simulink library "HEMERO"  (Simulink 3.00)
values from neighbouring files (symbols this model uses):
  K1 = 0.5    [ejh64.m]    (also in ejh65.m)
  K2 = 0.8    [ejh64.m]    (also in ejh65.m)
  x_camino = 0:0.01:10    [ejh64.m]    (also in ejh65.m)
  y_camino = x_camino.^2    [ejh64.m]    (also in ejh65.m)
undefined symbols (not defined in the file or in its folder): magnitude, nonlinear
libraries: simulink_extras x12, HEMERO x9, simulink3 x6, dspstat x4
(part 7 of 9)

== system HEMERO/Robots móviles/Control de robots móviles/Métodos basados en Teoría de Control/Seguimiento de caminos/Seguimiento de caminos (control no lineal)/Cálculo de parámetros/Cálculo de phi gorro/Subsystem2 ==
  fi_gorro : Inport  Port=1  PortWidth=-1  SampleTime=-1  DataType=auto
      settings: SignalType=auto
  Constant1 : Constant  Value=360
  Constant2 : Constant  Value=360
  Sum1 : Sum  Inputs=-+  SaturateOnIntegerOverflow=on
  Sum2 : Sum  Inputs=++  SaturateOnIntegerOverflow=on
  Switch : Switch  Threshold=180
  Switch1 : Switch  Threshold=0
  Switch2 : Switch  Threshold=-180
  fi_go_mo : Outport  Port=1
  wires:
  Constant2/1 -> Sum2/2
  fi_gorro/1 -> Sum2/1, Switch2/2, Switch2/1, Switch/2, Switch/3, Switch1/2, Sum1/2
  Sum2/1 -> Switch2/3
  Sum1/1 -> Switch/1
  Constant1/1 -> Sum1/1
  Switch2/1 -> Switch1/3
  Switch/1 -> Switch1/1
  Switch1/1 -> fi_go_mo/1

== system HEMERO/Robots móviles/Control de robots móviles/Métodos basados en Teoría de Control/Seguimiento de caminos/Seguimiento de caminos (control no lineal)/Cálculo de parámetros/Subsystem/Parametros de Curvatura ==
  x_1 : Inport  Port=1  PortWidth=-1  SampleTime=-1  DataType=auto
      settings: SignalType=auto
  x_2 : Inport  Port=2  PortWidth=-1  SampleTime=-1  DataType=auto
      settings: SignalType=auto
  x_3 : Inport  Port=3  PortWidth=-1  SampleTime=-1  DataType=auto
      settings: SignalType=auto
  y_1 : Inport  Port=4  PortWidth=-1  SampleTime=-1  DataType=auto
      settings: SignalType=auto
  y_2 : Inport  Port=5  PortWidth=-1  SampleTime=-1  DataType=auto
      settings: SignalType=auto
  y_3 : Inport  Port=6  PortWidth=-1  SampleTime=-1  DataType=auto
      settings: SignalType=auto
  Radio de  Curvatura : Subsystem
  coordenada x c. curvatura : Subsystem
  coordenada y c. curvatura : Subsystem
  x_g : Outport  Port=1  InitialOutput=0
  y_g : Outport  Port=2  InitialOutput=0
  R_c : Outport  Port=3  InitialOutput=0
  wires:
  y_3/1 -> coordenada x c. curvatura/6(y_3), coordenada y c. curvatura/6(y_3)
  y_2/1 -> coordenada y c. curvatura/5(y_2), coordenada x c. curvatura/5(y_2)
  y_1/1 -> Radio de  Curvatura/4(y_1), coordenada x c. curvatura/4(y_1), coordenada y c. curvatura/4(y_1)
  x_3/1 -> coordenada y c. curvatura/3(x_3), coordenada x c. curvatura/3(x_3)
  x_2/1 -> coordenada y c. curvatura/2(x_2), coordenada x c. curvatura/2(x_2)
  x_1/1 -> Radio de  Curvatura/2(x_1), coordenada y c. curvatura/1(x_1), coordenada x c. curvatura/1(x_1)
  coordenada x c. curvatura/1(x_g) -> Radio de  Curvatura/1(x_g), x_g/1
  coordenada y c. curvatura/1(y_g) -> Radio de  Curvatura/3(y_g), y_g/1
  Radio de  Curvatura/1(R_c) -> R_c/1

== system HEMERO/Robots móviles/Control de robots móviles/Métodos basados en Teoría de Control/Seguimiento de caminos/Seguimiento de caminos (control no lineal)/Cálculo de parámetros/Subsystem/Subsystem ==
  x : Inport  Port=1  PortWidth=-1  SampleTime=-1  DataType=auto
      settings: SignalType=auto
  y : Inport  Port=2  PortWidth=-1  SampleTime=-1  DataType=auto
      settings: SignalType=auto
  x_g : Inport  Port=3  PortWidth=-1  SampleTime=-1  DataType=auto
      settings: SignalType=auto
  y_g : Inport  Port=4  PortWidth=-1  SampleTime=-1  DataType=auto
      settings: SignalType=auto
  Math Function2 : Math  Operator=sqrt  OutputSignalType=auto
  Math Function3 : Math  Operator=square  OutputSignalType=auto
  Math Function4 : Math  Operator=square  OutputSignalType=auto
  Sum : Sum  Inputs=+-  SaturateOnIntegerOverflow=on
  Sum1 : Sum  Inputs=+-  SaturateOnIntegerOverflow=on
  Sum2 : Sum  Inputs=++  SaturateOnIntegerOverflow=on
  dist : Outport  Port=1  InitialOutput=0
  wires:
  Sum2/1 -> Math Function2/1
  Math Function4/1 -> Sum2/2
  Sum1/1 -> Math Function4/1
  Math Function3/1 -> Sum2/1
  Sum/1 -> Math Function3/1
  y/1 -> Sum1/1
  x_g/1 -> Sum/2
  x/1 -> Sum/1
  y_g/1 -> Sum1/2
  Math Function2/1 -> dist/1

== system HEMERO/Robots móviles/Control de robots móviles/Métodos basados en Teoría de Control/Seguimiento de caminos/Seguimiento de caminos (control no lineal)/Cálculo de parámetros/Subsystem/distancia mínima1 ==
  x_camino : Inport  Port=1  PortWidth=-1  SampleTime=-1  DataType=auto
      settings: SignalType=auto
  y_camino : Inport  Port=2  PortWidth=-1  SampleTime=-1  DataType=auto
      settings: SignalType=auto
  x_vehiculo : Inport  Port=3  PortWidth=-1  SampleTime=-1  DataType=auto
      settings: SignalType=auto
  y_vehiculo : Inport  Port=4  PortWidth=-1  SampleTime=-1  DataType=auto
      settings: SignalType=auto
  Math Function2 : Math  Operator=sqrt  OutputSignalType=auto
  Math Function3 : Math  Operator=square  OutputSignalType=auto
  Math Function4 : Math  Operator=square  OutputSignalType=auto
  Minimum : dspstat/Minimum
  Sum : Sum  Inputs=+-  SaturateOnIntegerOverflow=on
  Sum1 : Sum  Inputs=+-  SaturateOnIntegerOverflow=on
  Sum2 : Sum  Inputs=++  SaturateOnIntegerOverflow=on
  d_min : Outport  Port=1  InitialOutput=0
  indice : Outport  Port=2  InitialOutput=0
  wires:
  Minimum/2 -> indice/1
  Minimum/1 -> d_min/1
  Math Function2/1 -> Minimum/1
  Sum2/1 -> Math Function2/1
  Math Function4/1 -> Sum2/2
  Sum1/1 -> Math Function4/1
  Math Function3/1 -> Sum2/1
  Sum/1 -> Math Function3/1
  y_vehiculo/1 -> Sum1/2
  y_camino/1 -> Sum1/1
  x_vehiculo/1 -> Sum/2
  x_camino/1 -> Sum/1

== system HEMERO/Robots móviles/Control de robots móviles/Métodos basados en Teoría de Control/Seguimiento de caminos/Seguimiento de caminos (control no lineal)/Cálculo de parámetros/Subsystem/tres_puntos ==
  indice : Inport  Port=1  PortWidth=-1  SampleTime=-1  DataType=auto
      settings: SignalType=auto
  Constant : Constant  Value=1
  Constant1 : Constant  Value=2
  Look-Up Table : Lookup  InputValues=1:length(x_camino)  OutputValues=x_camino(1:length(x_camino))
  Look-Up Table1 : Lookup  InputValues=1:length(y_camino)  OutputValues=y_camino(1:length(y_camino))
  Look-Up Table2 : Lookup  InputValues=1:length(x_camino)  OutputValues=x_camino(1:length(x_camino))
  Look-Up Table3 : Lookup  InputValues=1:length(y_camino)  OutputValues=y_camino(1:length(y_camino))
  Look-Up Table4 : Lookup  InputValues=1:length(x_camino)  OutputValues=x_camino(1:length(x_camino))
  Look-Up Table5 : Lookup  InputValues=1:length(y_camino)  OutputValues=y_camino(1:length(y_camino))
  Sum : Sum  Inputs=++  SaturateOnIntegerOverflow=on
  Sum1 : Sum  Inputs=++  SaturateOnIntegerOverflow=on
  x_1 : Outport  Port=1
  x_2 : Outport  Port=2
  x_3 : Outport  Port=3
  y_1 : Outport  Port=4
  y_2 : Outport  Port=5
  y_3 : Outport  Port=6
  wires:
  Sum1/1 -> Look-Up Table5/1, Look-Up Table4/1
  Look-Up Table4/1 -> x_3/1
  Look-Up Table5/1 -> y_3/1
  Constant1/1 -> Sum1/2
  Look-Up Table1/1 -> y_1/1
  Sum/1 -> Look-Up Table3/1, Look-Up Table2/1
  Look-Up Table3/1 -> y_2/1
  Look-Up Table2/1 -> x_2/1
  Constant/1 -> Sum/2
  indice/1 -> Sum1/1, Sum/1, Look-Up Table1/1, Look-Up Table/1
  Look-Up Table/1 -> x_1/1

== system HEMERO/Robots móviles/Control de robots móviles/Métodos basados en Teoría de Control/Seguimiento de trayectorias/Ejemplos/Ejemplo H.6.6/Seguimiento de trayectorias (Control lineal)/Cambio de variable ==
  x_r : Inport  Port=1  PortWidth=-1  SampleTime=-1  DataType=auto
      settings: SignalType=auto
  x : Inport  Port=2  PortWidth=-1  SampleTime=-1  DataType=auto
      settings: SignalType=auto
  y_r : Inport  Port=3  PortWidth=-1  SampleTime=-1  DataType=auto
      settings: SignalType=auto
  y : Inport  Port=4  PortWidth=-1  SampleTime=-1  DataType=auto
      settings: SignalType=auto
  phi_r : Inport  Port=5  PortWidth=-1  SampleTime=-1  DataType=auto
      settings: SignalType=auto
  phi : Inport  Port=6  PortWidth=-1  SampleTime=-1  DataType=auto
      settings: SignalType=auto
  Cálculo de e1 : Subsystem
  Cálculo de e2 : Subsystem
  Cálculo de e3 : Subsystem
  e1 : Outport  Port=1
  e2 : Outport  Port=2
  e3 : Outport  Port=3
  wires:
  x_r/1 -> Cálculo de e1/1(x_r), Cálculo de e2/1(x_r)
  x/1 -> Cálculo de e1/2(x), Cálculo de e2/2(x)
  y_r/1 -> Cálculo de e1/3(y_r), Cálculo de e2/3(y_r)
  y/1 -> Cálculo de e1/4(y), Cálculo de e2/4(y)
  phi_r/1 -> Cálculo de e3/1(phi_r)
  phi/1 -> Cálculo de e2/5(phi), Cálculo de e3/2(phi), Cálculo de e1/5(phi)
  Cálculo de e1/1(e1) -> e1/1
  Cálculo de e2/1(e2) -> e2/1
  Cálculo de e3/1(e3) -> e3/1

== system HEMERO/Robots móviles/Control de robots móviles/Métodos basados en Teoría de Control/Seguimiento de trayectorias/Ejemplos/Ejemplo H.6.6/Seguimiento de trayectorias (Control lineal)/Configuración síncrona referencia ==
  v_r : Inport  Port=1  PortWidth=-1  SampleTime=-1  DataType=auto
      settings: SignalType=auto
  w_r : Inport  Port=2  PortWidth=-1  SampleTime=-1  DataType=auto
      settings: SignalType=auto
  Gain : Gain  Gain=-1  SaturateOnIntegerOverflow=on
  Integrator : Integrator  ExternalReset=none  InitialConditionSource=internal  InitialCondition=phi_r_inicial  LimitOutput=off  UpperSaturationLimit=inf  LowerSaturationLimit=-inf  ShowSaturationPort=off  ShowStatePort=off  AbsoluteTolerance=auto
  Integrator1 : Integrator  ExternalReset=none  InitialConditionSource=internal  InitialCondition=x_r_inicial  LimitOutput=off  UpperSaturationLimit=inf  LowerSaturationLimit=-inf  ShowSaturationPort=off  ShowStatePort=off  AbsoluteTolerance=auto
  Integrator2 : Integrator  ExternalReset=none  InitialConditionSource=internal  InitialCondition=y_r_inicial  LimitOutput=off  UpperSaturationLimit=inf  LowerSaturationLimit=-inf  ShowSaturationPort=off  ShowStatePort=off  AbsoluteTolerance=auto
  Product : Product  Inputs=2  SaturateOnIntegerOverflow=on
  Product1 : Product  Inputs=2  SaturateOnIntegerOverflow=on
  Trigonometric Function : Trigonometry  Operator=sin  OutputSignalType=auto
  Trigonometric Function1 : Trigonometry  Operator=cos  OutputSignalType=auto
  x_r : Outport  Port=1
  y_r : Outport  Port=2
  phi_r : Outport  Port=3
  wires:
  Product1/1 -> Integrator2/1
  Product/1 -> Integrator1/1
  Trigonometric Function1/1 -> Product1/2
  Integrator/1 -> Trigonometric Function1/1, Trigonometric Function/1, phi_r/1
  Integrator1/1 -> x_r/1
  Integrator2/1 -> y_r/1
  v_r/1 -> Product/1, Product1/1
  w_r/1 -> Integrator/1
  Trigonometric Function/1 -> Gain/1
  Gain/1 -> Product/2

== system HEMERO/Robots móviles/Control de robots móviles/Métodos basados en Teoría de Control/Seguimiento de trayectorias/Ejemplos/Ejemplo H.6.6/Seguimiento de trayectorias (Control lineal)/Configuración síncrona robot real ==
  v : Inport  Port=1  PortWidth=-1  SampleTime=-1  DataType=auto
      settings: SignalType=auto
  w : Inport  Port=2  PortWidth=-1  SampleTime=-1  DataType=auto
      settings: SignalType=auto
  Gain : Gain  Gain=-1  SaturateOnIntegerOverflow=on
  Integrator : Integrator  ExternalReset=none  InitialConditionSource=internal  InitialCondition=phi_inicial  LimitOutput=off  UpperSaturationLimit=inf  LowerSaturationLimit=-inf  ShowSaturationPort=off  ShowStatePort=off  AbsoluteTolerance=auto
  Integrator1 : Integrator  ExternalReset=none  InitialConditionSource=internal  InitialCondition=x_inicial  LimitOutput=off  UpperSaturationLimit=inf  LowerSaturationLimit=-inf  ShowSaturationPort=off  ShowStatePort=off  AbsoluteTolerance=auto
  Integrator2 : Integrator  ExternalReset=none  InitialConditionSource=internal  InitialCondition=y_inicial  LimitOutput=off  UpperSaturationLimit=inf  LowerSaturationLimit=-inf  ShowSaturationPort=off  ShowStatePort=off  AbsoluteTolerance=auto
  Product : Product  Inputs=2  SaturateOnIntegerOverflow=on
  Product1 : Product  Inputs=2  SaturateOnIntegerOverflow=on
  Trigonometric Function : Trigonometry  Operator=sin  OutputSignalType=auto
  Trigonometric Function1 : Trigonometry  Operator=cos  OutputSignalType=auto
  x : Outport  Port=1
  y : Outport  Port=2
  phi : Outport  Port=3
  wires:
  Product1/1 -> Integrator2/1
  Product/1 -> Integrator1/1
  Gain/1 -> Product/2
  Integrator/1 -> Trigonometric Function/1, Trigonometric Function1/1, phi/1
  Integrator1/1 -> x/1
  Integrator2/1 -> y/1
  v/1 -> Product/1, Product1/1
  w/1 -> Integrator/1
  Trigonometric Function/1 -> Gain/1
  Trigonometric Function1/1 -> Product1/2

== system HEMERO/Robots móviles/Control de robots móviles/Métodos basados en Teoría de Control/Seguimiento de trayectorias/Ejemplos/Ejemplo H.6.6/Seguimiento de trayectorias (Control lineal)/Control lineal ==
  e1 : Inport  Port=1  PortWidth=-1  SampleTime=-1  DataType=auto
      settings: SignalType=auto
  e2 : Inport  Port=2  PortWidth=-1  SampleTime=-1  DataType=auto
      settings: SignalType=auto
  e3 : Inport  Port=3  PortWidth=-1  SampleTime=-1  DataType=auto
      settings: SignalType=auto
  v_r : Inport  Port=4  PortWidth=-1  SampleTime=-1  DataType=auto
      settings: SignalType=auto
  Cálculo de u1 : Subsystem
  "Cálculo de u2 " : Subsystem
  u1 : Outport  Port=1
  u2 : Outport  Port=2
  wires:
  e1/1 -> Cálculo de u1/1(e1)
  e2/1 -> "Cálculo de u2 "/1(e2)
  e3/1 -> "Cálculo de u2 "/2(e3)
  Cálculo de u1/1(u1) -> u1/1
  "Cálculo de u2 "/1(u2) -> u2/1
  v_r/1 -> "Cálculo de u2 "/3(v_r)

== system HEMERO/Robots móviles/Control de robots móviles/Métodos basados en Teoría de Control/Seguimiento de trayectorias/Ejemplos/Ejemplo H.6.7/Seguimiento de trayectorias (Control lineal con escalado de velocidad)/Cambio de variable ==
  x_r : Inport  Port=1  PortWidth=-1  SampleTime=-1  DataType=auto
      settings: SignalType=auto
  x : Inport  Port=2  PortWidth=-1  SampleTime=-1  DataType=auto
      settings: SignalType=auto
  y_r : Inport  Port=3  PortWidth=-1  SampleTime=-1  DataType=auto
      settings: SignalType=auto
  y : Inport  Port=4  PortWidth=-1  SampleTime=-1  DataType=auto
      settings: SignalType=auto
  phi_r : Inport  Port=5  PortWidth=-1  SampleTime=-1  DataType=auto
      settings: SignalType=auto
  phi : Inport  Port=6  PortWidth=-1  SampleTime=-1  DataType=auto
      settings: SignalType=auto
  Cálculo de e1 : Subsystem
  Cálculo de e2 : Subsystem
  Cálculo de e3 : Subsystem
  e1 : Outport  Port=1
  e2 : Outport  Port=2
  e3 : Outport  Port=3
  wires:
  x_r/1 -> Cálculo de e1/1(x_r), Cálculo de e2/1(x_r)
  x/1 -> Cálculo de e1/2(x), Cálculo de e2/2(x)
  y_r/1 -> Cálculo de e1/3(y_r), Cálculo de e2/3(y_r)
  y/1 -> Cálculo de e1/4(y), Cálculo de e2/4(y)
  phi_r/1 -> Cálculo de e3/1(phi_r)
  phi/1 -> Cálculo de e2/5(phi), Cálculo de e3/2(phi), Cálculo de e1/5(phi)
  Cálculo de e1/1(e1) -> e1/1
  Cálculo de e2/1(e2) -> e2/1
  Cálculo de e3/1(e3) -> e3/1

== system HEMERO/Robots móviles/Control de robots móviles/Métodos basados en Teoría de Control/Seguimiento de trayectorias/Ejemplos/Ejemplo H.6.7/Seguimiento de trayectorias (Control lineal con escalado de velocidad)/Configuración síncrona referencia ==
  v_r : Inport  Port=1  PortWidth=-1  SampleTime=-1  DataType=auto
      settings: SignalType=auto
  w_r : Inport  Port=2  PortWidth=-1  SampleTime=-1  DataType=auto
      settings: SignalType=auto
  Gain : Gain  Gain=-1  SaturateOnIntegerOverflow=on
  Integrator : Integrator  ExternalReset=none  InitialConditionSource=internal  InitialCondition=phi_r_inicial  LimitOutput=off  UpperSaturationLimit=inf  LowerSaturationLimit=-inf  ShowSaturationPort=off  ShowStatePort=off  AbsoluteTolerance=auto
  Integrator1 : Integrator  ExternalReset=none  InitialConditionSource=internal  InitialCondition=x_r_inicial  LimitOutput=off  UpperSaturationLimit=inf  LowerSaturationLimit=-inf  ShowSaturationPort=off  ShowStatePort=off  AbsoluteTolerance=auto
  Integrator2 : Integrator  ExternalReset=none  InitialConditionSource=internal  InitialCondition=y_r_inicial  LimitOutput=off  UpperSaturationLimit=inf  LowerSaturationLimit=-inf  ShowSaturationPort=off  ShowStatePort=off  AbsoluteTolerance=auto
  Product : Product  Inputs=2  SaturateOnIntegerOverflow=on
  Product1 : Product  Inputs=2  SaturateOnIntegerOverflow=on
  Trigonometric Function : Trigonometry  Operator=sin  OutputSignalType=auto
  Trigonometric Function1 : Trigonometry  Operator=cos  OutputSignalType=auto
  x_r : Outport  Port=1
  y_r : Outport  Port=2
  phi_r : Outport  Port=3
  wires:
  Product1/1 -> Integrator2/1
  Product/1 -> Integrator1/1
  Gain/1 -> Product/2
  Integrator/1 -> Trigonometric Function/1, Trigonometric Function1/1, phi_r/1
  Integrator1/1 -> x_r/1
  Integrator2/1 -> y_r/1
  v_r/1 -> Product/1, Product1/1
  w_r/1 -> Integrator/1
  Trigonometric Function/1 -> Gain/1
  Trigonometric Function1/1 -> Product1/2

== system HEMERO/Robots móviles/Control de robots móviles/Métodos basados en Teoría de Control/Seguimiento de trayectorias/Ejemplos/Ejemplo H.6.7/Seguimiento de trayectorias (Control lineal con escalado de velocidad)/Configuración síncrona robot real ==
  v : Inport  Port=1  PortWidth=-1  SampleTime=-1  DataType=auto
      settings: SignalType=auto
  w : Inport  Port=2  PortWidth=-1  SampleTime=-1  DataType=auto
      settings: SignalType=auto
  Gain : Gain  Gain=-1  SaturateOnIntegerOverflow=on
  Integrator : Integrator  ExternalReset=none  InitialConditionSource=internal  InitialCondition=phi_inicial  LimitOutput=off  UpperSaturationLimit=inf  LowerSaturationLimit=-inf  ShowSaturationPort=off  ShowStatePort=off  AbsoluteTolerance=auto
  Integrator1 : Integrator  ExternalReset=none  InitialConditionSource=internal  InitialCondition=x_inicial  LimitOutput=off  UpperSaturationLimit=inf  LowerSaturationLimit=-inf  ShowSaturationPort=off  ShowStatePort=off  AbsoluteTolerance=auto
  Integrator2 : Integrator  ExternalReset=none  InitialConditionSource=internal  InitialCondition=y_inicial  LimitOutput=off  UpperSaturationLimit=inf  LowerSaturationLimit=-inf  ShowSaturationPort=off  ShowStatePort=off  AbsoluteTolerance=auto
  Product : Product  Inputs=2  SaturateOnIntegerOverflow=on
  Product1 : Product  Inputs=2  SaturateOnIntegerOverflow=on
  Trigonometric Function : Trigonometry  Operator=sin  OutputSignalType=auto
  Trigonometric Function1 : Trigonometry  Operator=cos  OutputSignalType=auto
  x : Outport  Port=1
  y : Outport  Port=2
  phi : Outport  Port=3
  wires:
  Product1/1 -> Integrator2/1
  Product/1 -> Integrator1/1
  Gain/1 -> Product/2
  Integrator/1 -> Trigonometric Function/1, Trigonometric Function1/1, phi/1
  Integrator1/1 -> x/1
  Integrator2/1 -> y/1
  v/1 -> Product/1, Product1/1
  w/1 -> Integrator/1
  Trigonometric Function/1 -> Gain/1
  Trigonometric Function1/1 -> Product1/2

== system HEMERO/Robots móviles/Control de robots móviles/Métodos basados en Teoría de Control/Seguimiento de trayectorias/Ejemplos/Ejemplo H.6.7/Seguimiento de trayectorias (Control lineal con escalado de velocidad)/Control lineal con escalado de velocidad ==
  e1 : Inport  Port=1  PortWidth=-1  SampleTime=-1  DataType=auto
      settings: SignalType=auto
  e2 : Inport  Port=2  PortWidth=-1  SampleTime=-1  DataType=auto
      settings: SignalType=auto
  e3 : Inport  Port=3  PortWidth=-1  SampleTime=-1  DataType=auto
      settings: SignalType=auto
  v_r : Inport  Port=4  PortWidth=-1  SampleTime=-1  DataType=auto
      settings: SignalType=auto
  w_r : Inport  Port=5  PortWidth=-1  SampleTime=-1  DataType=auto
      settings: SignalType=auto
  Cálculo de u1 : Subsystem
  "Cálculo de u2 " : Subsystem
  u1 : Outport  Port=1
  u2 : Outport  Port=2
  wires:
  e1/1 -> Cálculo de u1/1(e1)
  v_r/1 -> Cálculo de u1/2(v_r), "Cálculo de u2 "/3(v_r)
  e2/1 -> "Cálculo de u2 "/1(e2)
  e3/1 -> "Cálculo de u2 "/2(e3)
  Cálculo de u1/1(u1) -> u1/1
  "Cálculo de u2 "/1(u2) -> u2/1
  w_r/1 -> Cálculo de u1/3(w_r)
  Cálculo de u1/2(K1) -> "Cálculo de u2 "/4(K3)

== system HEMERO/Robots móviles/Control de robots móviles/Métodos basados en Teoría de Control/Seguimiento de trayectorias/Ejemplos/Ejemplo H.6.8/Seguimiento de trayectorias (Control no lineal)/Cambio de variable ==
  x_r : Inport  Port=1  PortWidth=-1  SampleTime=-1  DataType=auto
      settings: SignalType=auto
  x : Inport  Port=2  PortWidth=-1  SampleTime=-1  DataType=auto
      settings: SignalType=auto
  y_r : Inport  Port=3  PortWidth=-1  SampleTime=-1  DataType=auto
      settings: SignalType=auto
  y : Inport  Port=4  PortWidth=-1  SampleTime=-1  DataType=auto
      settings: SignalType=auto
  phi_r : Inport  Port=5  PortWidth=-1  SampleTime=-1  DataType=auto
      settings: SignalType=auto
  phi : Inport  Port=6  PortWidth=-1  SampleTime=-1  DataType=auto
      settings: SignalType=auto
  Cálculo de e1 : Subsystem
  Cálculo de e2 : Subsystem
  Cálculo de e3 : Subsystem
  e1 : Outport  Port=1
  e2 : Outport  Port=2
  e3 : Outport  Port=3
  wires:
  x_r/1 -> Cálculo de e1/1(x_r), Cálculo de e2/1(x_r)
  x/1 -> Cálculo de e1/2(x), Cálculo de e2/2(x)
  y_r/1 -> Cálculo de e1/3(y_r), Cálculo de e2/3(y_r)
  y/1 -> Cálculo de e1/4(y), Cálculo de e2/4(y)
  phi_r/1 -> Cálculo de e3/1(phi_r)
  phi/1 -> Cálculo de e2/5(phi), Cálculo de e3/2(phi), Cálculo de e1/5(phi)
  Cálculo de e1/1(e1) -> e1/1
  Cálculo de e2/1(e2) -> e2/1
  Cálculo de e3/1(e3) -> e3/1

== system HEMERO/Robots móviles/Control de robots móviles/Métodos basados en Teoría de Control/Seguimiento de trayectorias/Ejemplos/Ejemplo H.6.8/Seguimiento de trayectorias (Control no lineal)/Configuración síncrona referencia ==
  v_r : Inport  Port=1  PortWidth=-1  SampleTime=-1  DataType=auto
      settings: SignalType=auto
  w_r : Inport  Port=2  PortWidth=-1  SampleTime=-1  DataType=auto
      settings: SignalType=auto
  Gain : Gain  Gain=-1  SaturateOnIntegerOverflow=on
  Integrator : Integrator  ExternalReset=none  InitialConditionSource=internal  InitialCondition=phi_r_inicial  LimitOutput=off  UpperSaturationLimit=inf  LowerSaturationLimit=-inf  ShowSaturationPort=off  ShowStatePort=off  AbsoluteTolerance=auto
  Integrator1 : Integrator  ExternalReset=none  InitialConditionSource=internal  InitialCondition=x_r_inicial  LimitOutput=off  UpperSaturationLimit=inf  LowerSaturationLimit=-inf  ShowSaturationPort=off  ShowStatePort=off  AbsoluteTolerance=auto
  Integrator2 : Integrator  ExternalReset=none  InitialConditionSource=internal  InitialCondition=y_r_inicial  LimitOutput=off  UpperSaturationLimit=inf  LowerSaturationLimit=-inf  ShowSaturationPort=off  ShowStatePort=off  AbsoluteTolerance=auto
  Product : Product  Inputs=2  SaturateOnIntegerOverflow=on
  Product1 : Product  Inputs=2  SaturateOnIntegerOverflow=on
  Trigonometric Function : Trigonometry  Operator=sin  OutputSignalType=auto
  Trigonometric Function1 : Trigonometry  Operator=cos  OutputSignalType=auto
  x_r : Outport  Port=1
  y_r : Outport  Port=2
  phi_r : Outport  Port=3
  wires:
  Product1/1 -> Integrator2/1
  Product/1 -> Integrator1/1
  Integrator/1 -> Trigonometric Function/1, Trigonometric Function1/1, phi_r/1
  Integrator1/1 -> x_r/1
  Integrator2/1 -> y_r/1
  v_r/1 -> Product/1, Product1/1
  w_r/1 -> Integrator/1
  Gain/1 -> Product/2
  Trigonometric Function/1 -> Gain/1
  Trigonometric Function1/1 -> Product1/2

== system HEMERO/Robots móviles/Control de robots móviles/Métodos basados en Teoría de Control/Seguimiento de trayectorias/Ejemplos/Ejemplo H.6.8/Seguimiento de trayectorias (Control no lineal)/Configuración síncrona robot real ==
  v : Inport  Port=1  PortWidth=-1  SampleTime=-1  DataType=auto
      settings: SignalType=auto
  w : Inport  Port=2  PortWidth=-1  SampleTime=-1  DataType=auto
      settings: SignalType=auto
  Gain : Gain  Gain=-1  SaturateOnIntegerOverflow=on
  Integrator : Integrator  ExternalReset=none  InitialConditionSource=internal  InitialCondition=phi_inicial  LimitOutput=off  UpperSaturationLimit=inf  LowerSaturationLimit=-inf  ShowSaturationPort=off  ShowStatePort=off  AbsoluteTolerance=auto
  Integrator1 : Integrator  ExternalReset=none  InitialConditionSource=internal  InitialCondition=x_inicial  LimitOutput=off  UpperSaturationLimit=inf  LowerSaturationLimit=-inf  ShowSaturationPort=off  ShowStatePort=off  AbsoluteTolerance=auto
  Integrator2 : Integrator  ExternalReset=none  InitialConditionSource=internal  InitialCondition=y_inicial  LimitOutput=off  UpperSaturationLimit=inf  LowerSaturationLimit=-inf  ShowSaturationPort=off  ShowStatePort=off  AbsoluteTolerance=auto
  Product : Product  Inputs=2  SaturateOnIntegerOverflow=on
  Product1 : Product  Inputs=2  SaturateOnIntegerOverflow=on
  Trigonometric Function : Trigonometry  Operator=sin  OutputSignalType=auto
  Trigonometric Function1 : Trigonometry  Operator=cos  OutputSignalType=auto
  x : Outport  Port=1
  y : Outport  Port=2
  phi : Outport  Port=3
  wires:
  Product1/1 -> Integrator2/1
  Product/1 -> Integrator1/1
  Gain/1 -> Product/2
  Integrator/1 -> Trigonometric Function/1, Trigonometric Function1/1, phi/1
  Integrator1/1 -> x/1
  Integrator2/1 -> y/1
  v/1 -> Product/1, Product1/1
  w/1 -> Integrator/1
  Trigonometric Function/1 -> Gain/1
  Trigonometric Function1/1 -> Product1/2

== system HEMERO/Robots móviles/Control de robots móviles/Métodos basados en Teoría de Control/Seguimiento de trayectorias/Ejemplos/Ejemplo H.6.8/Seguimiento de trayectorias (Control no lineal)/Control no lineal ==
  e1 : Inport  Port=1  PortWidth=-1  SampleTime=-1  DataType=auto
      settings: SignalType=auto
  e2 : Inport  Port=2  PortWidth=-1  SampleTime=-1  DataType=auto
      settings: SignalType=auto
  e3 : Inport  Port=3  PortWidth=-1  SampleTime=-1  DataType=auto
      settings: SignalType=auto
  v_r : Inport  Port=4  PortWidth=-1  SampleTime=-1  DataType=auto
      settings: SignalType=auto
  K1 : Inport  Port=5  PortWidth=-1  SampleTime=-1  DataType=auto
      settings: SignalType=auto
  K3 : Inport  Port=6  PortWidth=-1  SampleTime=-1  DataType=auto
      settings: SignalType=auto
  Cálculo de u1 : Subsystem
  "Cálculo de u2 " : Subsystem
  u1 : Outport  Port=1
  u2 : Outport  Port=2
  wires:
  e1/1 -> Cálculo de u1/1(e1)
  e2/1 -> "Cálculo de u2 "/1(e2)
  e3/1 -> "Cálculo de u2 "/2(e3)
  Cálculo de u1/1(u1) -> u1/1
  "Cálculo de u2 "/1(u2) -> u2/1
  v_r/1 -> "Cálculo de u2 "/3(v_r)
  K1/1 -> Cálculo de u1/2(K1)
  K3/1 -> "Cálculo de u2 "/4(K3)

== system HEMERO/Robots móviles/Control de robots móviles/Métodos basados en Teoría de Control/Seguimiento de trayectorias/Ejemplos/Ejemplo H.6.8/Seguimiento de trayectorias (Control no lineal)/Cálculo de K1 y K3 ==
  w_r : Inport  Port=1  PortWidth=-1  SampleTime=-1  DataType=auto
      settings: SignalType=auto
  v_r : Inport  Port=2  PortWidth=-1  SampleTime=-1  DataType=auto
      settings: SignalType=auto
  Constant : Constant  Value=b
  Fcn : Fcn  Expr=u^2
  Fcn1 : Fcn  Expr=u^2
  Fcn2 : Fcn  Expr=sqrt(u)
  Gain1 : Gain  Gain=2*d  SaturateOnIntegerOverflow=on
  Product : Product  Inputs=2  SaturateOnIntegerOverflow=on
  Sum : Sum  Inputs=++  SaturateOnIntegerOverflow=on
  K1 : Outport  Port=1
  wires:
  w_r/1 -> Fcn/1
  v_r/1 -> Fcn1/1
  Fcn1/1 -> Product/1
  Constant/1 -> Product/2
  Product/1 -> Sum/1
  Fcn/1 -> Sum/2
  Sum/1 -> Fcn2/1
  Fcn2/1 -> Gain1/1
  Gain1/1 -> K1/1

== system HEMERO/Robots móviles/Control de robots móviles/Métodos basados en Teoría de Control/Seguimiento de trayectorias/Seguimiento de trayectorias (Control lineal con escalado de velocidad)/Cambio de variable/Cálculo de e3/Subsystem2 ==
  phi_gorro : Inport  Port=1  PortWidth=-1  SampleTime=-1  DataType=auto
      settings: SignalType=auto
  Constant1 : Constant  Value=360
  Constant2 : Constant  Value=360
  Sum1 : Sum  Inputs=-+  SaturateOnIntegerOverflow=on
  Sum2 : Sum  Inputs=++  SaturateOnIntegerOverflow=on
  Switch : Switch  Threshold=180
  Switch1 : Switch  Threshold=0
  Switch2 : Switch  Threshold=-180
  phi_go_mod : Outport  Port=1
  wires:
  Constant2/1 -> Sum2/2
  phi_gorro/1 -> Sum2/1, Switch2/2, Switch2/1, Switch/2, Switch/3, Switch1/2, Sum1/2
  Sum2/1 -> Switch2/3
  Sum1/1 -> Switch/1
  Constant1/1 -> Sum1/1
  Switch2/1 -> Switch1/3
  Switch/1 -> Switch1/1
  Switch1/1 -> phi_go_mod/1

== system HEMERO/Robots móviles/Control de robots móviles/Métodos basados en Teoría de Control/Seguimiento de trayectorias/Seguimiento de trayectorias (Control lineal)/Cambio de variable/Cálculo de e3/Subsystem2 ==
  phi_gorro : Inport  Port=1  PortWidth=-1  SampleTime=-1  DataType=auto
      settings: SignalType=auto
  Constant1 : Constant  Value=360
  Constant2 : Constant  Value=360
  Sum1 : Sum  Inputs=-+  SaturateOnIntegerOverflow=on
  Sum2 : Sum  Inputs=++  SaturateOnIntegerOverflow=on
  Switch : Switch  Threshold=180
  Switch1 : Switch  Threshold=0
  Switch2 : Switch  Threshold=-180
  phi_go_mod : Outport  Port=1
  wires:
  Constant2/1 -> Sum2/2
  phi_gorro/1 -> Sum2/1, Switch2/2, Switch2/1, Switch/2, Switch/3, Switch1/2, Sum1/2
  Sum2/1 -> Switch2/3
  Sum1/1 -> Switch/1
  Constant1/1 -> Sum1/1
  Switch2/1 -> Switch1/3
  Switch/1 -> Switch1/1
  Switch1/1 -> phi_go_mod/1

== system HEMERO/Robots móviles/Control de robots móviles/Métodos basados en Teoría de Control/Seguimiento de trayectorias/Seguimiento de trayectorias (Control no lineal)/Cambio de variable/Cálculo de e3/Subsystem2 ==
  phi_gorro : Inport  Port=1  PortWidth=-1  SampleTime=-1  DataType=auto
      settings: SignalType=auto
  Constant1 : Constant  Value=360
  Constant2 : Constant  Value=360
  Sum1 : Sum  Inputs=-+  SaturateOnIntegerOverflow=on
  Sum2 : Sum  Inputs=++  SaturateOnIntegerOverflow=on
  Switch : Switch  Threshold=180
  Switch1 : Switch  Threshold=0
  Switch2 : Switch  Threshold=-180
  phi_go_mod : Outport  Port=1
  wires:
  Constant2/1 -> Sum2/2
  phi_gorro/1 -> Sum2/1, Switch2/2, Switch2/1, Switch/2, Switch/3, Switch1/2, Sum1/2
  Sum2/1 -> Switch2/3
  Sum1/1 -> Switch/1
  Constant1/1 -> Sum1/1
  Switch2/1 -> Switch1/3
  Switch/1 -> Switch1/1
  Switch1/1 -> phi_go_mod/1

== system HEMERO/Robots móviles/Control de robots móviles/Métodos basados en Teoría de Control/Seguimiento de caminos/Ejemplos/Ejemplo H.6.4/Seguimiento de caminos (control lineal)/Cálculo de parámetros/Cálculo de phi gorro ==
  fi_vehiculo : Inport  Port=1  PortWidth=-1  SampleTime=-1  DataType=auto
      settings: SignalType=auto
  indice : Inport  Port=2  PortWidth=-1  SampleTime=-1  DataType=auto
      settings: SignalType=auto
  Subsystem : Subsystem
      mask Type: Pasa phi a un ángulo entre -180 y 180
      mask Description: Pasa phi a un ángulo entre -180 y 180
      mask Help: Pasa phi a un ángulo entre -180 y 180
  Subsystem1 : Subsystem
  Subsystem2 : Subsystem
      mask Description: Pasa phi gorro al intervalo -180,180
  suma : Sum  Inputs=+-  SaturateOnIntegerOverflow=on
  fi_go_mo : Outport  Port=1
  wires:
  Subsystem2/1(fi_go_mo) -> fi_go_mo/1
  suma/1 -> Subsystem2/1(fi_gorro)
  Subsystem/1(fi_veh_mod) -> suma/1
  indice/1 -> Subsystem1/1(indice)
  fi_vehiculo/1 -> Subsystem/1(fi_vehiculo)
  Subsystem1/1(fi_camino) -> suma/2

== system HEMERO/Robots móviles/Control de robots móviles/Métodos basados en Teoría de Control/Seguimiento de caminos/Ejemplos/Ejemplo H.6.4/Seguimiento de caminos (control lineal)/Cálculo de parámetros/Subsystem ==
  x_camino : Inport  Port=1  PortWidth=-1  SampleTime=-1  DataType=auto
      settings: SignalType=auto
  y_camino : Inport  Port=2  PortWidth=-1  SampleTime=-1  DataType=auto
      settings: SignalType=auto
  x_vehiculo : Inport  Port=3  PortWidth=-1  SampleTime=-1  DataType=auto
      settings: SignalType=auto
  y_vehiculo : Inport  Port=4  PortWidth=-1  SampleTime=-1  DataType=auto
      settings: SignalType=auto
  Parametros de Curvatura : Subsystem
  Product : Product  Inputs=2  SaturateOnIntegerOverflow=on
  Rc - dist : Sum  Inputs=-+  SaturateOnIntegerOverflow=on
  Sign : Signum
  Subsystem : Subsystem
  distancia mínima1 : Subsystem
  tres_puntos : Subsystem
  distancia : Outport  Port=1
  indice : Outport  Port=2
  R_c : Outport  Port=3
  wires:
  distancia mínima1/2(indice) -> tres_puntos/1(indice), indice/1
  Parametros de Curvatura/3(R_c) -> R_c/1, Rc - dist/2
  y_vehiculo/1 -> Subsystem/2(y), distancia mínima1/4(y_vehiculo)
  x_vehiculo/1 -> Subsystem/1(x), distancia mínima1/3(x_vehiculo)
  tres_puntos/4(y_1) -> Parametros de Curvatura/4(y_1)
  tres_puntos/1(x_1) -> Parametros de Curvatura/1(x_1)
  Product/1 -> distancia/1
  y_camino/1 -> distancia mínima1/2(y_camino)
  x_camino/1 -> distancia mínima1/1(x_camino)
  tres_puntos/6(y_3) -> Parametros de Curvatura/6(y_3)
  tres_puntos/5(y_2) -> Parametros de Curvatura/5(y_2)
  tres_puntos/3(x_3) -> Parametros de Curvatura/3(x_3)
  tres_puntos/2(x_2) -> Parametros de Curvatura/2(x_2)
  distancia mínima1/1(d_min) -> Product/2
  Sign/1 -> Product/1
  Parametros de Curvatura/1(x_g) -> Subsystem/3(x_g)
  Parametros de Curvatura/2(y_g) -> Subsystem/4(y_g)
  Subsystem/1(dist) -> Rc - dist/1
  Rc - dist/1 -> Sign/1

== system HEMERO/Robots móviles/Control de robots móviles/Métodos basados en Teoría de Control/Seguimiento de caminos/Ejemplos/Ejemplo H.6.5/Seguimiento de caminos (control no lineal)/Cálculo de parámetros/Cálculo de phi gorro ==
  fi_vehiculo : Inport  Port=1  PortWidth=-1  SampleTime=-1  DataType=auto
      settings: SignalType=auto
  indice : Inport  Port=2  PortWidth=-1  SampleTime=-1  DataType=auto
      settings: SignalType=auto
  Subsystem : Subsystem
      mask Type: Pasa phi a un ángulo entre -180 y 180
      mask Description: Pasa phi a un ángulo entre -180 y 180
      mask Help: Pasa phi a un ángulo entre -180 y 180
  Subsystem1 : Subsystem
  Subsystem2 : Subsystem
      mask Description: Pasa phi gorro al intervalo -180,180
  suma : Sum  Inputs=+-  SaturateOnIntegerOverflow=on
  fi_go_mo : Outport  Port=1
  wires:
  Subsystem2/1(fi_go_mo) -> fi_go_mo/1
  suma/1 -> Subsystem2/1(fi_gorro)
  Subsystem/1(fi_veh_mod) -> suma/1
  indice/1 -> Subsystem1/1(indice)
  fi_vehiculo/1 -> Subsystem/1(fi_vehiculo)
  Subsystem1/1(fi_camino) -> suma/2

== system HEMERO/Robots móviles/Control de robots móviles/Métodos basados en Teoría de Control/Seguimiento de caminos/Ejemplos/Ejemplo H.6.5/Seguimiento de caminos (control no lineal)/Cálculo de parámetros/Subsystem ==
  x_camino : Inport  Port=1  PortWidth=-1  SampleTime=-1  DataType=auto
      settings: SignalType=auto
  y_camino : Inport  Port=2  PortWidth=-1  SampleTime=-1  DataType=auto
      settings: SignalType=auto
  x_vehiculo : Inport  Port=3  PortWidth=-1  SampleTime=-1  DataType=auto
      settings: SignalType=auto
  y_vehiculo : Inport  Port=4  PortWidth=-1  SampleTime=-1  DataType=auto
      settings: SignalType=auto
  Parametros de Curvatura : Subsystem
  Product : Product  Inputs=2  SaturateOnIntegerOverflow=on
  Rc - dist : Sum  Inputs=-+  SaturateOnIntegerOverflow=on
  Sign : Signum
  Subsystem : Subsystem
  distancia mínima1 : Subsystem
  tres_puntos : Subsystem
  distancia : Outport  Port=1
  indice : Outport  Port=2
  R_c : Outport  Port=3
  wires:
  distancia mínima1/2(indice) -> tres_puntos/1(indice), indice/1
  Parametros de Curvatura/3(R_c) -> R_c/1, Rc - dist/2
  y_vehiculo/1 -> Subsystem/2(y), distancia mínima1/4(y_vehiculo)
  x_vehiculo/1 -> Subsystem/1(x), distancia mínima1/3(x_vehiculo)
  tres_puntos/4(y_1) -> Parametros de Curvatura/4(y_1)
  tres_puntos/1(x_1) -> Parametros de Curvatura/1(x_1)
  Product/1 -> distancia/1
  y_camino/1 -> distancia mínima1/2(y_camino)
  x_camino/1 -> distancia mínima1/1(x_camino)
  tres_puntos/6(y_3) -> Parametros de Curvatura/6(y_3)
  tres_puntos/5(y_2) -> Parametros de Curvatura/5(y_2)
  tres_puntos/3(x_3) -> Parametros de Curvatura/3(x_3)
  tres_puntos/2(x_2) -> Parametros de Curvatura/2(x_2)
  distancia mínima1/1(d_min) -> Product/2
  Sign/1 -> Product/1
  Parametros de Curvatura/1(x_g) -> Subsystem/3(x_g)
  Parametros de Curvatura/2(y_g) -> Subsystem/4(y_g)
  Subsystem/1(dist) -> Rc - dist/1
  Rc - dist/1 -> Sign/1

== system HEMERO/Robots móviles/Control de robots móviles/Métodos basados en Teoría de Control/Seguimiento de caminos/Seguimiento de caminos (control lineal)/Cálculo de parámetros/Subsystem/Parametros de Curvatura/Radio de  Curvatura ==
  x_g : Inport  Port=1  PortWidth=-1  SampleTime=-1  DataType=auto
      settings: SignalType=auto
  x_1 : Inport  Port=2  PortWidth=-1  SampleTime=-1  DataType=auto
      settings: SignalType=auto
  y_g : Inport  Port=3  PortWidth=-1  SampleTime=-1  DataType=auto
      settings: SignalType=auto
  y_1 : Inport  Port=4  PortWidth=-1  SampleTime=-1  DataType=auto
      settings: SignalType=auto
  Math Function : Math  Operator=square  OutputSignalType=auto
  Math Function1 : Math  Operator=sqrt  OutputSignalType=auto
  Math Function2 : Math  Operator=square  OutputSignalType=auto
  Sum : Sum  Inputs=+-  SaturateOnIntegerOverflow=on
  Sum1 : Sum  Inputs=+-  SaturateOnIntegerOverflow=on
  Sum2 : Sum  Inputs=++  SaturateOnIntegerOverflow=on
  R_c : Outport  Port=1  InitialOutput=0
  wires:
  x_g/1 -> Sum/2
  x_1/1 -> Sum/1
  y_1/1 -> Sum1/1
  y_g/1 -> Sum1/2
  Sum/1 -> Math Function/1
  Sum1/1 -> Math Function2/1
  Math Function/1 -> Sum2/1
  Math Function2/1 -> Sum2/2
  Sum2/1 -> Math Function1/1
  Math Function1/1 -> R_c/1

== system HEMERO/Robots móviles/Control de robots móviles/Métodos basados en Teoría de Control/Seguimiento de caminos/Seguimiento de caminos (control lineal)/Cálculo de parámetros/Subsystem/Parametros de Curvatura/coordenada x c. curvatura ==
  x_1 : Inport  Port=1  PortWidth=-1  SampleTime=-1  DataType=auto
      settings: SignalType=auto
  x_2 : Inport  Port=2  PortWidth=-1  SampleTime=-1  DataType=auto
      settings: SignalType=auto
  x_3 : Inport  Port=3  PortWidth=-1  SampleTime=-1  DataType=auto
      settings: SignalType=auto
  y_1 : Inport  Port=4  PortWidth=-1  SampleTime=-1  DataType=auto
      settings: SignalType=auto
  y_2 : Inport  Port=5  PortWidth=-1  SampleTime=-1  DataType=auto
      settings: SignalType=auto
  y_3 : Inport  Port=6  PortWidth=-1  SampleTime=-1  DataType=auto
      settings: SignalType=auto
  Constant : Constant  Value=0.00000001
  Math Function : Math  Operator=reciprocal  OutputSignalType=auto
  Product{,1..4} (5 alike) : Product  Inputs=2  SaturateOnIntegerOverflow=on
  Sum : Sum  Inputs=+-  SaturateOnIntegerOverflow=on
  Sum1 : Sum  Inputs=+-  SaturateOnIntegerOverflow=on
  Switch : Switch  Threshold=0.00000001
  bloque_1 : Subsystem
  bloque_2 : Subsystem
  x_g : Outport  Port=1  InitialOutput=0
  wires:
  Sum/1 -> Product4/1
  y_3/1 -> bloque_2/4(y3)
  y_2/1 -> bloque_1/4(y2), bloque_2/3(y2)
  x_3/1 -> bloque_2/2(x3)
  y_1/1 -> bloque_1/3(y1)
  x_2/1 -> bloque_2/1(x2), bloque_1/2(x2)
  x_1/1 -> bloque_1/1(x1)
  bloque_2/1(alfa_2) -> Product3/2
  bloque_1/2(beta_1) -> Product3/1, Product1/1
  bloque_1/1(alfa_1) -> Product2/1
  bloque_2/2(beta_2) -> Product2/2, Product/1
  bloque_2/3(c_2) -> Product1/2
  bloque_1/3(c_1) -> Product/2
  Math Function/1 -> Product4/2
  Product3/1 -> Sum1/2
  Product2/1 -> Sum1/1
  Product1/1 -> Sum/2
  Product/1 -> Sum/1
  Product4/1 -> x_g/1
  Sum1/1 -> Switch/2, Switch/1
  Constant/1 -> Switch/3
  Switch/1 -> Math Function/1

== system HEMERO/Robots móviles/Control de robots móviles/Métodos basados en Teoría de Control/Seguimiento de caminos/Seguimiento de caminos (control lineal)/Cálculo de parámetros/Subsystem/Parametros de Curvatura/coordenada y c. curvatura ==
  x_1 : Inport  Port=1  PortWidth=-1  SampleTime=-1  DataType=auto
      settings: SignalType=auto
  x_2 : Inport  Port=2  PortWidth=-1  SampleTime=-1  DataType=auto
      settings: SignalType=auto
  x_3 : Inport  Port=3  PortWidth=-1  SampleTime=-1  DataType=auto
      settings: SignalType=auto
  y_1 : Inport  Port=4  PortWidth=-1  SampleTime=-1  DataType=auto
      settings: SignalType=auto
  y_2 : Inport  Port=5  PortWidth=-1  SampleTime=-1  DataType=auto
      settings: SignalType=auto
  y_3 : Inport  Port=6  PortWidth=-1  SampleTime=-1  DataType=auto
      settings: SignalType=auto
  Constant : Constant  Value=0.00000001
  Math Function : Math  Operator=reciprocal  OutputSignalType=auto
  Product{,1..4} (5 alike) : Product  Inputs=2  SaturateOnIntegerOverflow=on
  Sum : Sum  Inputs=+-  SaturateOnIntegerOverflow=on
  Sum1 : Sum  Inputs=+-  SaturateOnIntegerOverflow=on
  Switch : Switch  Threshold=0.00000001
  bloque_1 : Subsystem
  bloque_2 : Subsystem
  y_g : Outport  Port=1  InitialOutput=0
  wires:
  Sum/1 -> Product4/1
  y_3/1 -> bloque_2/4(y3)
  y_2/1 -> bloque_1/4(y2), bloque_2/3(y2)
  x_3/1 -> bloque_2/2(x3)
  y_1/1 -> bloque_1/3(y1)
  x_2/1 -> bloque_2/1(x2), bloque_1/2(x2)
  x_1/1 -> bloque_1/1(x1)
  Product3/1 -> Sum1/2
  Product2/1 -> Sum1/1
  Product1/1 -> Sum/2
  Product/1 -> Sum/1
  bloque_2/1(alfa_2) -> Product3/1, Product1/2
  bloque_1/2(beta_1) -> Product3/2
  bloque_2/2(beta_2) -> Product2/2
  bloque_1/1(alfa_1) -> Product2/1, Product/1
  bloque_1/3(c_1) -> Product1/1
  bloque_2/3(c_2) -> Product/2
  Product4/1 -> y_g/1
  Math Function/1 -> Product4/2
  Switch/1 -> Math Function/1
  Sum1/1 -> Switch/2, Switch/1
  Constant/1 -> Switch/3

== system HEMERO/Robots móviles/Control de robots móviles/Métodos basados en Teoría de Control/Seguimiento de caminos/Seguimiento de caminos (control no lineal)/Cálculo de parámetros/Subsystem/Parametros de Curvatura/Radio de  Curvatura ==
  x_g : Inport  Port=1  PortWidth=-1  SampleTime=-1  DataType=auto
      settings: SignalType=auto
  x_1 : Inport  Port=2  PortWidth=-1  SampleTime=-1  DataType=auto
      settings: SignalType=auto
  y_g : Inport  Port=3  PortWidth=-1  SampleTime=-1  DataType=auto
      settings: SignalType=auto
  y_1 : Inport  Port=4  PortWidth=-1  SampleTime=-1  DataType=auto
      settings: SignalType=auto
  Math Function : Math  Operator=square  OutputSignalType=auto
  Math Function1 : Math  Operator=sqrt  OutputSignalType=auto
  Math Function2 : Math  Operator=square  OutputSignalType=auto
  Sum : Sum  Inputs=+-  SaturateOnIntegerOverflow=on
  Sum1 : Sum  Inputs=+-  SaturateOnIntegerOverflow=on
  Sum2 : Sum  Inputs=++  SaturateOnIntegerOverflow=on
  R_c : Outport  Port=1  InitialOutput=0
  wires:
  Math Function1/1 -> R_c/1
  Sum2/1 -> Math Function1/1
  Math Function2/1 -> Sum2/2
  Math Function/1 -> Sum2/1
  Sum1/1 -> Math Function2/1
  Sum/1 -> Math Function/1
  y_g/1 -> Sum1/2
  y_1/1 -> Sum1/1
  x_1/1 -> Sum/1
  x_g/1 -> Sum/2

== system HEMERO/Robots móviles/Control de robots móviles/Métodos basados en Teoría de Control/Seguimiento de caminos/Seguimiento de caminos (control no lineal)/Cálculo de parámetros/Subsystem/Parametros de Curvatura/coordenada x c. curvatura ==
  x_1 : Inport  Port=1  PortWidth=-1  SampleTime=-1  DataType=auto
      settings: SignalType=auto
  x_2 : Inport  Port=2  PortWidth=-1  SampleTime=-1  DataType=auto
      settings: SignalType=auto
  x_3 : Inport  Port=3  PortWidth=-1  SampleTime=-1  DataType=auto
      settings: SignalType=auto
  y_1 : Inport  Port=4  PortWidth=-1  SampleTime=-1  DataType=auto
      settings: SignalType=auto
  y_2 : Inport  Port=5  PortWidth=-1  SampleTime=-1  DataType=auto
      settings: SignalType=auto
  y_3 : Inport  Port=6  PortWidth=-1  SampleTime=-1  DataType=auto
      settings: SignalType=auto
  Constant : Constant  Value=0.00000001
  Math Function : Math  Operator=reciprocal  OutputSignalType=auto
  Product{,1..4} (5 alike) : Product  Inputs=2  SaturateOnIntegerOverflow=on
  Sum : Sum  Inputs=+-  SaturateOnIntegerOverflow=on
  Sum1 : Sum  Inputs=+-  SaturateOnIntegerOverflow=on
  Switch : Switch  Threshold=0.00000001
  bloque_1 : Subsystem
  bloque_2 : Subsystem
  x_g : Outport  Port=1  InitialOutput=0
  wires:
  Switch/1 -> Math Function/1
  Constant/1 -> Switch/3
  Sum1/1 -> Switch/1, Switch/2
  Product4/1 -> x_g/1
  Product/1 -> Sum/1
  Product1/1 -> Sum/2
  Product2/1 -> Sum1/1
  Product3/1 -> Sum1/2
  Math Function/1 -> Product4/2
  bloque_1/3(c_1) -> Product/2
  bloque_2/3(c_2) -> Product1/2
  bloque_2/2(beta_2) -> Product/1, Product2/2
  bloque_1/1(alfa_1) -> Product2/1
  bloque_1/2(beta_1) -> Product1/1, Product3/1
  bloque_2/1(alfa_2) -> Product3/2
  x_1/1 -> bloque_1/1(x1)
  x_2/1 -> bloque_1/2(x2), bloque_2/1(x2)
  y_1/1 -> bloque_1/3(y1)
  x_3/1 -> bloque_2/2(x3)
  y_2/1 -> bloque_2/3(y2), bloque_1/4(y2)
  y_3/1 -> bloque_2/4(y3)
  Sum/1 -> Product4/1

== system HEMERO/Robots móviles/Control de robots móviles/Métodos basados en Teoría de Control/Seguimiento de caminos/Seguimiento de caminos (control no lineal)/Cálculo de parámetros/Subsystem/Parametros de Curvatura/coordenada y c. curvatura ==
  x_1 : Inport  Port=1  PortWidth=-1  SampleTime=-1  DataType=auto
      settings: SignalType=auto
  x_2 : Inport  Port=2  PortWidth=-1  SampleTime=-1  DataType=auto
      settings: SignalType=auto
  x_3 : Inport  Port=3  PortWidth=-1  SampleTime=-1  DataType=auto
      settings: SignalType=auto
  y_1 : Inport  Port=4  PortWidth=-1  SampleTime=-1  DataType=auto
      settings: SignalType=auto
  y_2 : Inport  Port=5  PortWidth=-1  SampleTime=-1  DataType=auto
      settings: SignalType=auto
  y_3 : Inport  Port=6  PortWidth=-1  SampleTime=-1  DataType=auto
      settings: SignalType=auto
  Constant : Constant  Value=0.00000001
  Math Function : Math  Operator=reciprocal  OutputSignalType=auto
  Product{,1..4} (5 alike) : Product  Inputs=2  SaturateOnIntegerOverflow=on
  Sum : Sum  Inputs=+-  SaturateOnIntegerOverflow=on
  Sum1 : Sum  Inputs=+-  SaturateOnIntegerOverflow=on
  Switch : Switch  Threshold=0.00000001
  bloque_1 : Subsystem
  bloque_2 : Subsystem
  y_g : Outport  Port=1  InitialOutput=0
  wires:
  Constant/1 -> Switch/3
  Sum1/1 -> Switch/1, Switch/2
  Switch/1 -> Math Function/1
  Math Function/1 -> Product4/2
  Product4/1 -> y_g/1
  bloque_2/3(c_2) -> Product/2
  bloque_1/3(c_1) -> Product1/1
  bloque_1/1(alfa_1) -> Product/1, Product2/1
  bloque_2/2(beta_2) -> Product2/2
  bloque_1/2(beta_1) -> Product3/2
  bloque_2/1(alfa_2) -> Product1/2, Product3/1
  Product/1 -> Sum/1
  Product1/1 -> Sum/2
  Product2/1 -> Sum1/1
  Product3/1 -> Sum1/2
  x_1/1 -> bloque_1/1(x1)
  x_2/1 -> bloque_1/2(x2), bloque_2/1(x2)
  y_1/1 -> bloque_1/3(y1)
  x_3/1 -> bloque_2/2(x3)
  y_2/1 -> bloque_2/3(y2), bloque_1/4(y2)
  y_3/1 -> bloque_2/4(y3)
  Sum/1 -> Product4/1

== system HEMERO/Robots móviles/Control de robots móviles/Métodos basados en Teoría de Control/Seguimiento de trayectorias/Ejemplos/Ejemplo H.6.6/Seguimiento de trayectorias (Control lineal)/Cambio de variable/Cálculo de e1 ==
  x_r : Inport  Port=1  PortWidth=-1  SampleTime=-1  DataType=auto
      settings: SignalType=auto
  x : Inport  Port=2  PortWidth=-1  SampleTime=-1  DataType=auto
      settings: SignalType=auto
  y_r : Inport  Port=3  PortWidth=-1  SampleTime=-1  DataType=auto
      settings: SignalType=auto
  y : Inport  Port=4  PortWidth=-1  SampleTime=-1  DataType=auto
      settings: SignalType=auto
  phi : Inport  Port=5  PortWidth=-1  SampleTime=-1  DataType=auto
      settings: SignalType=auto
  Product : Product  Inputs=2  SaturateOnIntegerOverflow=on
  Product1 : Product  Inputs=2  SaturateOnIntegerOverflow=on
  Sum : Sum  Inputs=-+  SaturateOnIntegerOverflow=on
  Sum1 : Sum  Inputs=+-  SaturateOnIntegerOverflow=on
  Sum2 : Sum  Inputs=++  SaturateOnIntegerOverflow=on
  Trigonometric Function : Trigonometry  Operator=sin  OutputSignalType=auto
  Trigonometric Function1 : Trigonometry  Operator=cos  OutputSignalType=auto
  e1 : Outport  Port=1
  wires:
  x_r/1 -> Sum/1
  x/1 -> Sum/2
  y_r/1 -> Sum1/1
  y/1 -> Sum1/2
  phi/1 -> Trigonometric Function/1, Trigonometric Function1/1
  Sum/1 -> Product/1
  Trigonometric Function/1 -> Product/2
  Sum1/1 -> Product1/1
  Trigonometric Function1/1 -> Product1/2
  Product/1 -> Sum2/1
  Product1/1 -> Sum2/2
  Sum2/1 -> e1/1

== system HEMERO/Robots móviles/Control de robots móviles/Métodos basados en Teoría de Control/Seguimiento de trayectorias/Ejemplos/Ejemplo H.6.6/Seguimiento de trayectorias (Control lineal)/Cambio de variable/Cálculo de e2 ==
  x_r : Inport  Port=1  PortWidth=-1  SampleTime=-1  DataType=auto
      settings: SignalType=auto
  x : Inport  Port=2  PortWidth=-1  SampleTime=-1  DataType=auto
      settings: SignalType=auto
  y_r : Inport  Port=3  PortWidth=-1  SampleTime=-1  DataType=auto
      settings: SignalType=auto
  y : Inport  Port=4  PortWidth=-1  SampleTime=-1  DataType=auto
      settings: SignalType=auto
  phi : Inport  Port=5  PortWidth=-1  SampleTime=-1  DataType=auto
      settings: SignalType=auto
  Product : Product  Inputs=2  SaturateOnIntegerOverflow=on
  Product1 : Product  Inputs=2  SaturateOnIntegerOverflow=on
  Sum : Sum  Inputs=-+  SaturateOnIntegerOverflow=on
  Sum1 : Sum  Inputs=-+  SaturateOnIntegerOverflow=on
  Sum2 : Sum  Inputs=++  SaturateOnIntegerOverflow=on
  Trigonometric Function2 : Trigonometry  Operator=sin  OutputSignalType=auto
  Trigonometric Function3 : Trigonometry  Operator=cos  OutputSignalType=auto
  e2 : Outport  Port=1
  wires:
  x_r/1 -> Sum/1
  x/1 -> Sum/2
  y_r/1 -> Sum1/1
  y/1 -> Sum1/2
  phi/1 -> Trigonometric Function3/1, Trigonometric Function2/1
  Sum/1 -> Product/1
  Trigonometric Function3/1 -> Product/2
  Sum1/1 -> Product1/1
  Trigonometric Function2/1 -> Product1/2
  Product/1 -> Sum2/1
  Product1/1 -> Sum2/2
  Sum2/1 -> e2/1

== system HEMERO/Robots móviles/Control de robots móviles/Métodos basados en Teoría de Control/Seguimiento de trayectorias/Ejemplos/Ejemplo H.6.6/Seguimiento de trayectorias (Control lineal)/Cambio de variable/Cálculo de e3 ==
  phi_r : Inport  Port=1  PortWidth=-1  SampleTime=-1  DataType=auto
      settings: SignalType=auto
  phi : Inport  Port=2  PortWidth=-1  SampleTime=-1  DataType=auto
      settings: SignalType=auto
  Subsystem2 : Subsystem
      mask Description: Pasa phi gorro al intervalo -180,180
  suma : Sum  Inputs=+-  SaturateOnIntegerOverflow=on
  e3 : Outport  Port=1
  wires:
  phi/1 -> suma/2
  phi_r/1 -> suma/1
  suma/1 -> Subsystem2/1(phi_gorro)
  Subsystem2/1(phi_go_mod) -> e3/1
